simulink model "LAB1_4_real"  (R2025b)
settings: Solver=ode3  StartTime=0.0  StopTime=10  FixedStep=0.001  RelTol=1e-3
undefined symbols (not defined in the file or in its folder): degs2rpm, delta_c, den_Hi, k_z0, k_z1, k_z2, k_zx, mot, National_Instruments, num_Hi, PCI, rpm2rads, sens, w0, w_c
libraries: sldrtlib x3
settings Model: SimulationMode=external  ExtModeTrigDuration=100001  Creator=delpratogi  LastModifiedBy=Simone
settings DataIOCC: ReturnWorkspaceOutputs=off
settings HardwareCC: ProdBitPerLong=64.0  ProdHWDeviceType=Intel->x86-64 (Linux 64)
settings RTWCC: SystemTargetFile=sldrt.tlc  TemplateMakefile=sldrt.tmf  RTWCompilerOptimization=on  Description=Simulink Desktop Real-Time
settings CodeAppCC: MaxIdLength=95.0
settings STFCustomTargetCC: SystemTargetFile=sldrt.tlc  TargetLangStandard=C99 (ISO)  ModelReferenceCompliant=off  ConcurrentExecutionCompliant=off  MATLABClassNameForMDSCustomization=Simulink.SoftwareTarget.TargetSpecificTriggerConfigurationBase

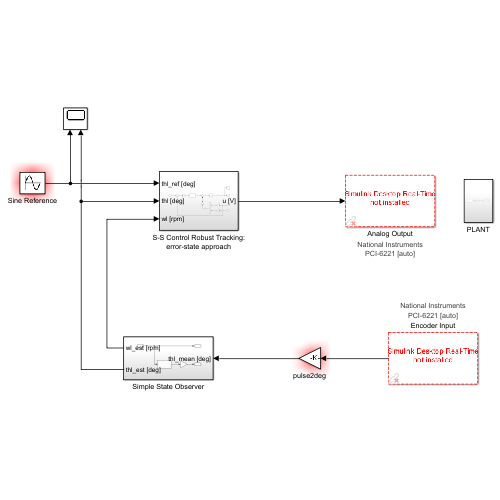
[thumbnail: Simulink's stored preview of the top-level diagram]
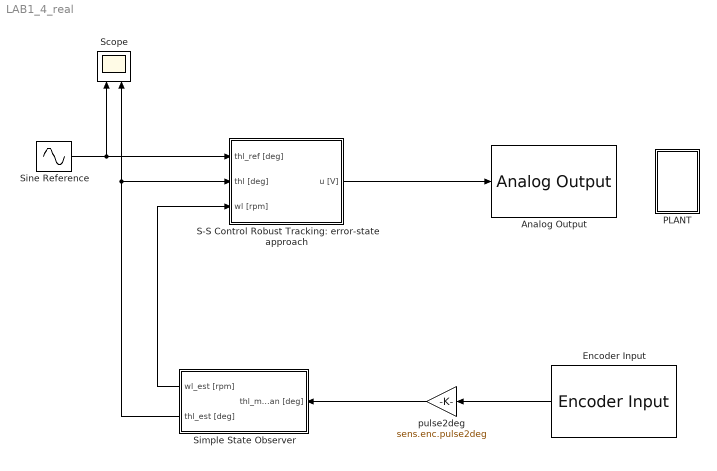
== system LAB1_4_real ==
  Analog Output : sldrtlib/Analog Output  SampleTime=0.001  MaxMissedTicks=10  ShowMissedTicks=off  YieldWhenWaiting=off  DrvName=National_Instruments/PCI-6221  DrvAddress=4294967295  DrvOptions=[0 0 0 2 0]  Channels=1  RangeMode=1  VoltRange=1  InitialValue=0  FinalValue=0
      settings: AttributesFormatString=National Instruments\nPCI-6221 [auto]
  Encoder Input : sldrtlib/Encoder Input  SampleTime=0.001  MaxMissedTicks=10  ShowMissedTicks=off  YieldWhenWaiting=off  DrvName=National_Instruments/PCI-6221  DrvAddress=4294967295  DrvOptions=[0 0 0 2 0]  Channels=1  QuadMode=3  IndexPulse=1  InputFilter=Inf  DataType=1
      settings: AttributesFormatString=National Instruments\nPCI-6221 [auto]
  PLANT : Subsystem
  S-S Control Robust Tracking: error-state approach : Subsystem
  Scope : Scope  NumInputPorts=2
      settings: ActiveDisplayYMinimum=-27.9225  ActiveDisplayYMaximum=29.9025
  Simple State Observer : Subsystem
  Sine Reference : Sin  Amplitude=20  Frequency=w0  SampleTime=0
  pulse2deg : Gain  Gain=sens.enc.pulse2deg
  wires:
  Encoder Input/1 -> pulse2deg/1
  S-S Control Robust Tracking: error-state approach/1(u [V]) -> Analog Output/1
  pulse2deg/1 -> Simple State Observer/1(thl_mean [deg])
  Simple State Observer/2(thl_est [deg]) -> S-S Control Robust Tracking: error-state approach/2(thl [deg]), Scope/2
  Simple State Observer/1(wl_est [rpm]) -> S-S Control Robust Tracking: error-state approach/3(wl [rpm])
  Sine Reference/1 -> S-S Control Robust Tracking: error-state approach/1(thl_ref [deg]), Scope/1

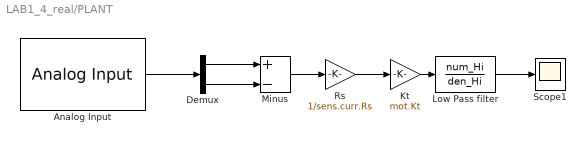
== system LAB1_4_real/PLANT ==
  Analog Input : sldrtlib/Analog Input  SampleTime=0.001  MaxMissedTicks=10  ShowMissedTicks=off  YieldWhenWaiting=off  DrvName=National_Instruments/PCI-6221  DrvAddress=4294967295  DrvOptions=[0 0 0 2 0]  Channels=[1,2]  RangeMode=1  VoltRange=1  DataType=1
      settings: AttributesFormatString=National Instruments\nPCI-6221 [auto]
  Demux : Demux  Outputs=2
  Kt : Gain  Gain=mot.Kt
  Low Pass filter : TransferFcn  Numerator=num_Hi  Denominator=den_Hi
  Minus : Sum  Inputs=+-
  Rs : Gain  Gain=1/sens.curr.Rs
  Scope1 : Scope
  wires:
  Low Pass filter/1 -> Scope1/1
  Demux/1 -> Minus/1
  Minus/1 -> Rs/1
  Analog Input/1 -> Demux/1
  Kt/1 -> Low Pass filter/1
  Demux/2 -> Minus/2
  Rs/1 -> Kt/1

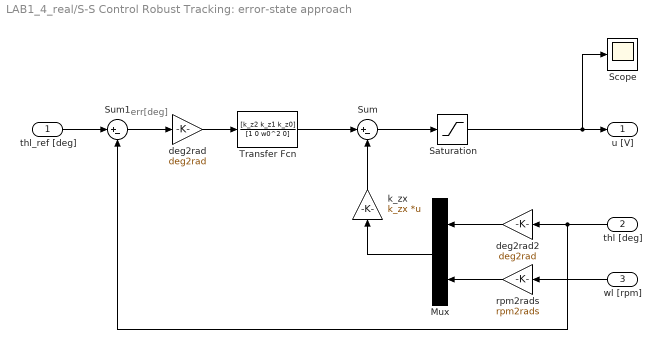
== system LAB1_4_real/S-S Control Robust Tracking: error-state approach ==
  note: err[deg]
  thl_ref [deg] : Inport
  thl [deg] : Inport  Port=2
  wl [rpm] : Inport  Port=3
  Mux : Mux  Inputs=2
  Saturation : Saturate  UpperLimit=10  LowerLimit=-10  ZeroCross=off
  Scope : Scope
      settings: ActiveDisplayYMinimum=-12.5  ActiveDisplayYMaximum=12.5  DataLoggingVariableName=ScopeData2
  Sum : Sum  Inputs=|+-
  Sum1 : Sum  Inputs=|+-
  Transfer Fcn : TransferFcn  Numerator=[k_z2 k_z1 k_z0]  Denominator=[1 0 w0^2 0]
  deg2rad : Gain  Gain=deg2rad
  deg2rad2 : Gain  Gain=deg2rad
  k_zx : Gain  Gain=k_zx  Multiplication=Matrix(K*u)
  rpm2rads : Gain  Gain=rpm2rads
  u [V] : Outport
  wires:
  deg2rad2/1 -> Mux/1
  rpm2rads/1 -> Mux/2
  Saturation/1 -> Scope/1, u [V]/1
  thl [deg]/1 -> Sum1/2, deg2rad2/1
  wl [rpm]/1 -> rpm2rads/1
  Mux/1 -> k_zx/1
  k_zx/1 -> Sum/2
  Sum/1 -> Saturation/1
  deg2rad/1 -> Transfer Fcn/1
  Transfer Fcn/1 -> Sum/1
  thl_ref [deg]/1 -> Sum1/1
  Sum1/1 -> deg2rad/1

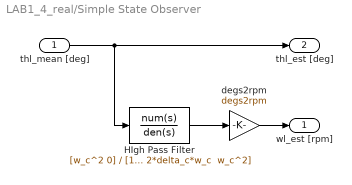
== system LAB1_4_real/Simple State Observer ==
  thl_mean [deg] : Inport
  HIgh Pass Filter : TransferFcn  Numerator=[w_c^2 0]  Denominator="[1 2*delta_c*w_c  w_c^2]"
  degs2rpm : Gain  Gain=degs2rpm
  wl_est [rpm] : Outport
  thl_est [deg] : Outport  Port=2
  wires:
  thl_mean [deg]/1 -> HIgh Pass Filter/1, thl_est [deg]/1
  HIgh Pass Filter/1 -> degs2rpm/1
  degs2rpm/1 -> wl_est [rpm]/1
